simulink model "quad_sim_mult_UAVs_coop_localization"  (R2017a)
settings: Solver=VariableStepAuto  StartTime=0.0  StopTime=60  FixedStep=0.02  MaxStep=0.03  MinStep=0.02  RelTol=1e-3  EnableMultiTasking=on
InitFcn:
  | setup_gains
  | % --- Outer loop gains --------
  | %P_X=9.44;   I_X=0.23;  D_X=2.36;
  | %P_Y=9.33;   I_Y=0.18;  D_Y=1.54;
  | % --------------------------
  | 
  | %CARLA TUNNED PID
  | %P_Z = 51.037;       I_Z = 43.051;        D_Z = 11.771;
  | %P_Z = 0.5;       I_Z = 0.15;        D_Z = 0.2;
  | %P_Z = 32.55;       I_Z = 9.82;        D_Z = 4.65 ;
  | 
  | global clientID;
  | clientID=-1;
values from neighbouring files (symbols this model uses):
  End_POS_coop = Start_POS+0.5    [setup_gains.m]
  Kd_az = 0.001    [setup_gains.m]
  Kd_px = 0.5    [setup_gains.m]
  Kd_py = 0.5    [setup_gains.m]
  Kd_pz = 0.025    [setup_gains.m]
  Kd_vx = 2    [setup_gains.m]
  Kd_vy = 2    [setup_gains.m]
  Kd_vz = 0.05    [setup_gains.m]
  Ki_az = 0.01    [setup_gains.m]
  Ki_px = 0.001    [setup_gains.m]
  Ki_py = 0.001    [setup_gains.m]
  Ki_pz = 0.001    [setup_gains.m]
  Ki_vx = 0.1    [setup_gains.m]
  Ki_vy = 0.1    [setup_gains.m]
  Ki_vz = 2.5    [setup_gains.m]
  Kp_az = 0.75    [setup_gains.m]
  Kp_px = 1    [setup_gains.m]
  Kp_py = 1    [setup_gains.m]
  Kp_pz = 0.5    [setup_gains.m]
  Kp_vx = 15.00    (= 15)    [setup_gains.m]
  Kp_vy = 15.00    (= 15)    [setup_gains.m]
  Kp_vz = 5    [setup_gains.m]
  s1 = cputime()*10    [setup_gains.m]
  s2 = round(s1+randn*10 + 1)    [setup_gains.m]
  s3 = round(s2+randn*10 + 32)    [setup_gains.m]
  s4 = round(s3+randn*10 + 55)    [setup_gains.m]
  Start_POS = [ -1.00 -1.00 1.05 ... (first row only)    [setup_gains.m]
  var_accel = 0.0001    [setup_gains.m]
  var_pos = 0.5^2    (= 0.25)    [setup_gains.m]
  var_ranges = 0.0025    [setup_gains.m]
undefined symbols (not defined in the file or in its folder): W, X, Y, Z
libraries: dspindex x15, robotlib x13, dspsigops x12
(part 1 of 2)
settings Model: Creator=kleber  LastModifiedBy=Cabral
settings DataIOCC: SaveFormat=Array
settings OptimizationCC: LifeSpan=inf
settings DebuggingCC: SolverPrmCheckMsg=warning  SFUnexpectedBacktrackingDiag=warning  SFNoUnconditionalDefaultTransitionDiag=warning  SFExecutionAtInitializationDiag=none
settings HardwareCC: ProdBitPerPointer=32  ProdBitPerSizeT=32  ProdBitPerPtrDiffT=32  ProdLargestAtomicFloat=None  ProdIntDivRoundTo=Undefined  ProdEndianess=Unspecified  ProdWordSize=32  ProdHWDeviceType=32-bit Generic
settings ModelReferenceCC: PropagateSignalLabelsOutOfModel=off
settings GRTTargetCC: TargetLangStandard=C89/C90 (ANSI)  GeneratePreprocessorConditionals=Disable all
settings ConfigComp: CovMetricSettings=dw  CovHtmlReporting=on  CovSaveCumulativeToWorkspaceVar=on  CovSaveSingleToWorkspaceVar=on  CovExternalEMLEnable=off  CovSFcnEnable=off

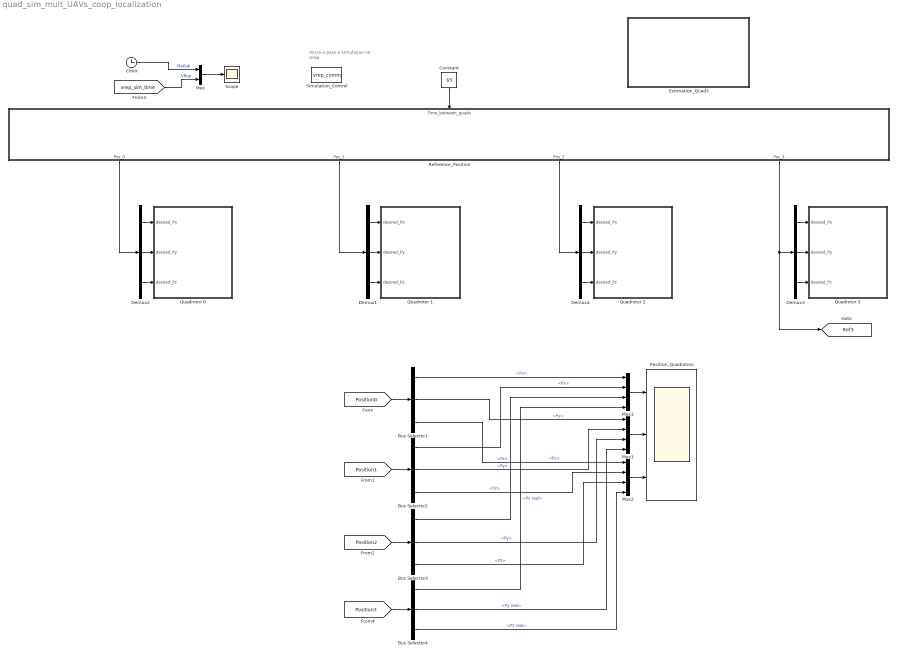
== system quad_sim_mult_UAVs_coop_localization ==
  note: Inicia e para a simulaçao no Vrep
  Bus Selector1 : BusSelector  OutputSignals=Px,Py,Pz
  Bus Selector2 : BusSelector  OutputSignals=Px,Py,Pz
  Bus Selector3 : BusSelector  OutputSignals=Px,Py,Pz
  Bus Selector4 : BusSelector  OutputSignals=Px real,Py real,Pz real
  Clock : Clock
  Constant : Constant  Value=65
  Demux{1..4} (4 alike) : Demux  Outputs=3
  Estimation_Quad3 : Subsystem
  Mux : Mux  Inputs=2
  Mux1 : Mux
  Mux2 : Mux
  Mux3 : Mux
  Position_Quadrotors : Scope  NumInputPorts=3
  Quadrotor 0 : Subsystem
  Quadrotor 1 : Subsystem
  Quadrotor 2 : Subsystem
  Quadrotor 3 : Subsystem
  Reference_Position : Subsystem
  Scope : Scope
  Simulation_Control : S-Function  FunctionName=vrep_comm  SFunctionDeploymentMode=off  EnableBusSupport=off
  tag scope: Ref3=global
  wires:
  Constant/1 -> Reference_Position/1(Time_between_quads)
  Demux1/1 -> Quadrotor 1/1(desired_Px)
  Demux1/2 -> Quadrotor 1/2(desired_Py)
  Demux1/3 -> Quadrotor 1/3(desired_Pz)
  Demux2/1 -> Quadrotor 0/1(desired_Px)
  Demux2/2 -> Quadrotor 0/2(desired_Py)
  Demux2/3 -> Quadrotor 0/3(desired_Pz)
  Reference_Position/1(Pos_0) -> Demux2/1
  Reference_Position/2(Pos_1) -> Demux1/1
  Demux4/1 -> Quadrotor 2/1(desired_Px)
  Demux4/2 -> Quadrotor 2/2(desired_Py)
  Demux4/3 -> Quadrotor 2/3(desired_Pz)
  Reference_Position/3(Pos_2) -> Demux4/1
  Demux3/1 -> Quadrotor 3/1(desired_Px)
  Demux3/2 -> Quadrotor 3/2(desired_Py)
  Demux3/3 -> Quadrotor 3/3(desired_Pz)
  Reference_Position/4(Pos_3) -> [Ref3], Demux3/1
  Mux/1 -> Scope/1
  Clock/1 -> Mux/1  "Matlab"
  [vrep_sim_time] -> Mux/2  "VRep"
  Bus Selector1/1 -> Mux3/1  "<Px>"
  [Position0] -> Bus Selector1/1
  Bus Selector1/2 -> Mux1/1  "<Py>"
  Bus Selector1/3 -> Mux2/1  "<Pz>"
  [Position1] -> Bus Selector2/1
  Bus Selector2/3 -> Mux2/2  "<Pz>"
  Bus Selector2/2 -> Mux1/2  "<Py>"
  Bus Selector2/1 -> Mux3/2  "<Px>"
  [Position2] -> Bus Selector3/1
  Bus Selector3/2 -> Mux1/3  "<Py>"
  Bus Selector3/3 -> Mux2/3  "<Pz>"
  Bus Selector3/1 -> Mux3/3  "<Px>"
  [Position3] -> Bus Selector4/1
  Mux3/1 -> Position_Quadrotors/1
  Mux2/1 -> Position_Quadrotors/3
  Mux1/1 -> Position_Quadrotors/2
  Bus Selector4/1 -> Mux3/4  "<Px real>"
  Bus Selector4/2 -> Mux1/4  "<Py real>"
  Bus Selector4/3 -> Mux2/4  "<Pz real>"

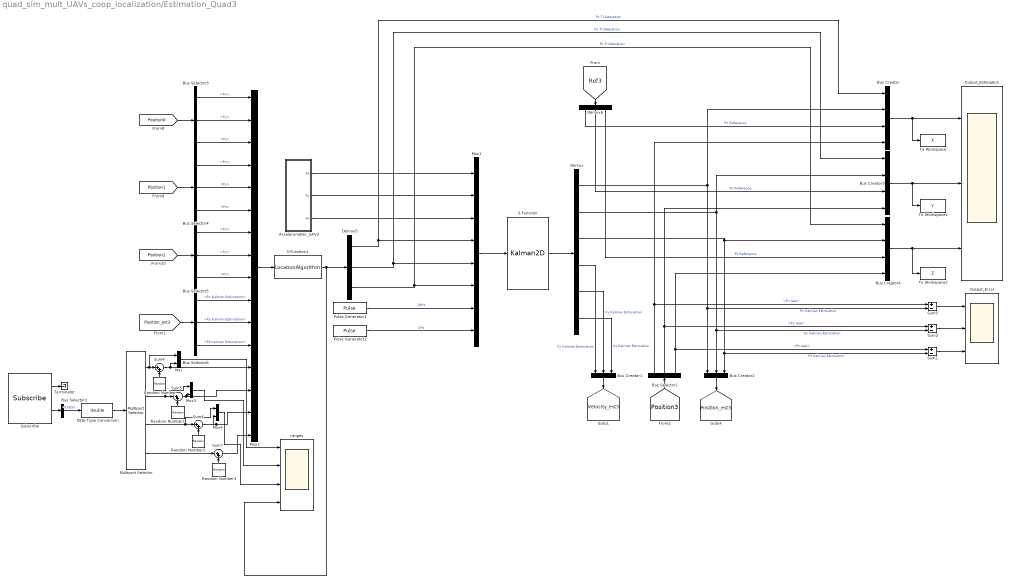
== system quad_sim_mult_UAVs_coop_localization/Estimation_Quad3 ==
  Accelerometer_UAV3 : Subsystem
  Bus Creator : BusCreator  Inputs=4
  Bus Creator1 : BusCreator  Inputs=3
  Bus Creator2 : BusCreator  Inputs=3
  Bus Creator3 : BusCreator  Inputs=4
  Bus Creator4 : BusCreator  Inputs=4
  Bus Selector1 : BusSelector  OutputSignals=Px real,Py real,Pz real
  Bus Selector2 : BusSelector  OutputSignals=Data
  Bus Selector3 : BusSelector  OutputSignals=Px,Py,Pz
  Bus Selector4 : BusSelector  OutputSignals=Px,Py,Pz
  Bus Selector5 : BusSelector  OutputSignals=Px,Py,Pz
  Bus Selector6 : BusSelector  OutputSignals=Px Kalman Estimation,Py Kalman Estimation,Pz Kalman Estimation
  Data Type Conversion : DataTypeConversion  OutDataTypeStr=double
  Demux : Demux  Outputs=6
  Demux5 : Demux  Outputs=3
  Demux6 : Demux  Outputs=3
  Multiport Selector : dspindex/Multiport Selector  rowsOrCols=Rows  idxCellArray={ 3,5,6,7}  idxErrMode=Generate Error
  Mux : Mux  Inputs=2
  Mux1 : Mux  Inputs=8
  Mux2 : Mux  Inputs=16
  Mux3 : Mux  Inputs=2
  Mux4 : Mux  Inputs=2
  Output_Error : Scope  NumInputPorts=3
  Output_Estimation : Scope  NumInputPorts=3
  Pulse Generator1 : DiscretePulseGenerator  PulseType=Time based  Period=0.1  PulseWidth=50
  Pulse Generator2 : DiscretePulseGenerator  PulseType=Time based  Period=1  PulseWidth=50
  Random Number : RandomNumber  Variance=var_ranges  Seed=s1  SampleTime=0.1
  Random Number1 : RandomNumber  Variance=var_ranges  Seed=s2  SampleTime=0.1
  Random Number2 : RandomNumber  Variance=var_ranges  Seed=s3  SampleTime=0.1
  Random Number3 : RandomNumber  Variance=var_ranges  Seed=s4  SampleTime=0.1
  S-Function : S-Function  FunctionName=Kalman2D  SFunctionDeploymentMode=off  EnableBusSupport=off
  S-Function1 : S-Function  FunctionName=LocationAlgorithm  SFunctionDeploymentMode=off  EnableBusSupport=off
  Subscribe : robotlib/Subscribe  SourceLibraryInfo=This block requires Robotics System Toolbox  topicSource=Select from ROS network  topic=/RangeSensors  messageType=std_msgs/Float32MultiArray  sampleTime=-1  messageQueueLength=51
      settings: SourceProductBaseCode=RO
  Sum1 : Sum  Inputs=+-
  Sum2 : Sum  Inputs=+-
  Sum3 : Sum  Inputs=+-
  Sum{4..7} (4 alike) : Sum  Inputs=|++
  Terminator : Terminator
  To Workspace : ToWorkspace  VariableName=X  SaveFormat=Timeseries  SampleTime=-1
  To Workspace1 : ToWorkspace  VariableName=Y  SaveFormat=Timeseries  SampleTime=-1
  To Workspace2 : ToWorkspace  VariableName=Z  SaveFormat=Timeseries  SampleTime=-1
  ranges : Scope  NumInputPorts=4
  tag scope: Position_est3=global, Velocity_est3=global
  wires:
  Bus Selector4/2 -> Mux2/5  "<Py>"
  Multiport Selector/4 -> Sum7/1
  Bus Selector5/3 -> Mux2/9  "<Pz>"
  [Position1] -> Bus Selector4/1
  Random Number3/1 -> Sum7/2
  Random Number/1 -> Sum4/2
  Random Number2/1 -> Sum6/2
  Subscribe/1 -> Terminator/1
  Sum4/1 -> Mux/2, Mux2/13
  Multiport Selector/2 -> Mux3/1, Sum5/1
  Sum5/1 -> Mux3/2, Mux2/14
  Mux2/1 -> S-Function1/1
  Multiport Selector/1 -> Mux/1, Sum4/1
  Bus Selector5/1 -> Mux2/7  "<Px>"
  Bus Selector5/2 -> Mux2/8  "<Py>"
  Sum6/1 -> Mux4/2, Mux2/15
  [Position2] -> Bus Selector5/1
  Random Number1/1 -> Sum5/2
  Bus Selector4/1 -> Mux2/4  "<Px>"
  Bus Selector4/3 -> Mux2/6  "<Pz>"
  Subscribe/2 -> Bus Selector2/1
  S-Function1/1 -> Demux5/1, ranges/4
  Bus Selector3/3 -> Mux2/3  "<Pz>"
  Bus Selector3/2 -> Mux2/2  "<Py>"
  Multiport Selector/3 -> Mux4/1, Sum6/1
  Bus Selector3/1 -> Mux2/1  "<Px>"
  Data Type Conversion/1 -> Multiport Selector/1
  Sum7/1 -> Mux2/16
  Bus Selector2/1 -> Data Type Conversion/1  "<Data>"
  [Position0] -> Bus Selector3/1
  Demux5/2 -> Mux1/5, Bus Creator3/1  "Py Trilateration"
  Demux/1 -> Bus Creator/2, Sum3/2, Bus Creator2/1  "Px Kalman Estimation"
  Demux/2 -> Bus Creator3/2, Sum2/2, Bus Creator2/2  "Py Kalman Estimation"
  Bus Creator/1 -> To Workspace/1, Output_Estimation/1
  Pulse Generator1/1 -> Mux1/7  "10Hz"
  Bus Creator3/1 -> Output_Estimation/2, To Workspace1/1
  Bus Creator4/1 -> To Workspace2/1, Output_Estimation/3
  S-Function/1 -> Demux/1
  Demux5/1 -> Bus Creator/1, Mux1/4  "Px Trilateration"
  Mux1/1 -> S-Function/1
  Pulse Generator2/1 -> Mux1/8  "1Hz"
  Demux5/3 -> Bus Creator4/1, Mux1/6  "Pz Trilateration"
  Demux/3 -> Sum1/2, Bus Creator2/3, Bus Creator4/2  "Pz Kalman Estimation"
  [Position3] -> Bus Selector1/1
  Bus Selector1/1 -> Sum3/1, Bus Creator/4  "<Px real>"
  Bus Selector1/2 -> Bus Creator3/4, Sum2/1  "<Py real>"
  Bus Selector1/3 -> Bus Creator4/4, Sum1/1  "<Pz real>"
  [Ref3] -> Demux6/1
  Demux6/1 -> Bus Creator/3  "Px Reference"
  Demux6/2 -> Bus Creator3/3  "Py Reference"
  Demux6/3 -> Bus Creator4/3  "Pz Reference"
  Bus Creator2/1 -> [Position_est3]
  Accelerometer_UAV3/2(Ay) -> Mux1/2
  Accelerometer_UAV3/3(Az) -> Mux1/3
  Accelerometer_UAV3/1(Ax) -> Mux1/1
  Sum3/1 -> Output_Error/1
  Sum2/1 -> Output_Error/2
  Sum1/1 -> Output_Error/3
  Bus Creator1/1 -> [Velocity_est3]
  Demux/6 -> Bus Creator1/3  "Vz Kalman Estimation"
  Demux/5 -> Bus Creator1/2  "Vy Kalman Estimation"
  Demux/4 -> Bus Creator1/1  "Vx Kalman Estimation"
  Mux4/1 -> ranges/3
  Mux3/1 -> ranges/2
  Mux/1 -> ranges/1
  Bus Selector6/1 -> Mux2/10  "<Px Kalman Estimation>"
  Bus Selector6/2 -> Mux2/11  "<Py Kalman Estimation>"
  Bus Selector6/3 -> Mux2/12  "<Pz Kalman Estimation>"
  [Position_est3] -> Bus Selector6/1

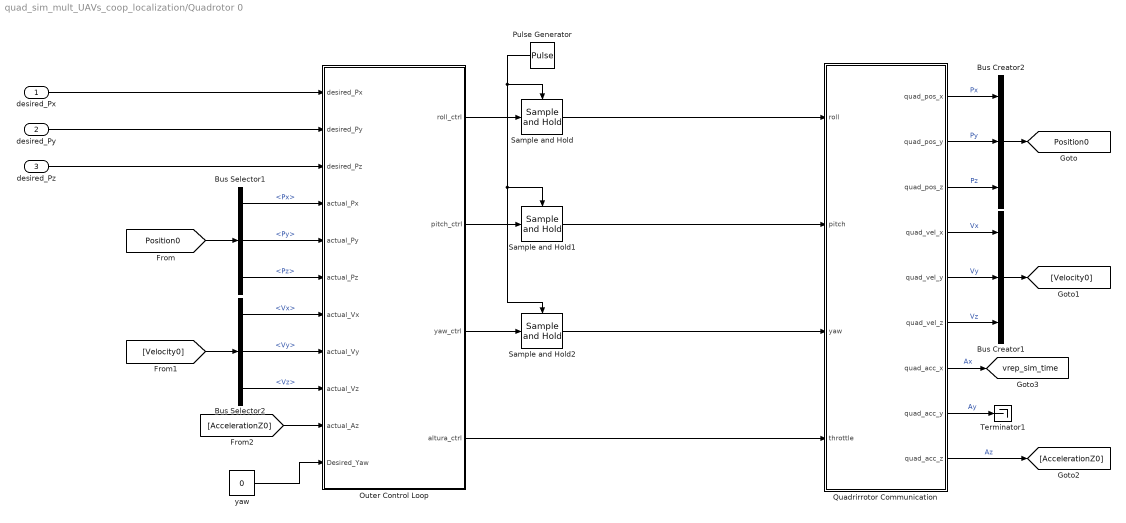
== system quad_sim_mult_UAVs_coop_localization/Quadrotor 0 ==
  desired_Px : Inport
  desired_Py : Inport  Port=2
  desired_Pz : Inport  Port=3
  Bus Creator1 : BusCreator  Inputs=3
  Bus Creator2 : BusCreator  Inputs=3
  Bus Selector1 : BusSelector  OutputSignals=Px,Py,Pz
  Bus Selector2 : BusSelector  OutputSignals=Vx,Vy,Vz
  Outer Control Loop : Subsystem
  Pulse Generator : DiscretePulseGenerator  PulseType=Time based  Period=0.1  PulseWidth=20
  Quadrirrotor Communication : Subsystem
  Sample and Hold : dspsigops/Sample and Hold  trig=Rising edge  initCond=0  latchinput=off
  Sample and Hold1 : dspsigops/Sample and Hold  trig=Rising edge  initCond=0  latchinput=off
  Sample and Hold2 : dspsigops/Sample and Hold  trig=Rising edge  initCond=0  latchinput=off
  Terminator1 : Terminator
  yaw : Constant  Value=0
  tag scope: Position0=global, vrep_sim_time=global
  wires:
  Quadrirrotor Communication/8(quad_acc_y) -> Terminator1/1  "Ay"
  [AccelerationZ0] -> Outer Control Loop/10(actual_Az)
  Quadrirrotor Communication/9(quad_acc_z) -> [AccelerationZ0]  "Az"
  yaw/1 -> Outer Control Loop/11(Desired_Yaw)
  Pulse Generator/1 -> Sample and Hold/Trigger, Sample and Hold1/Trigger, Sample and Hold2/Trigger
  Outer Control Loop/3(yaw_ctrl) -> Sample and Hold2/1
  Outer Control Loop/2(pitch_ctrl) -> Sample and Hold1/1
  Outer Control Loop/1(roll_ctrl) -> Sample and Hold/1
  desired_Py/1 -> Outer Control Loop/2(desired_Py)
  desired_Px/1 -> Outer Control Loop/1(desired_Px)
  desired_Pz/1 -> Outer Control Loop/3(desired_Pz)
  [Position0] -> Bus Selector1/1
  Bus Selector1/3 -> Outer Control Loop/6(actual_Pz)  "<Pz>"
  Bus Selector1/2 -> Outer Control Loop/5(actual_Py)  "<Py>"
  Bus Selector1/1 -> Outer Control Loop/4(actual_Px)  "<Px>"
  Quadrirrotor Communication/4(quad_vel_x) -> Bus Creator1/1  "Vx"
  Quadrirrotor Communication/5(quad_vel_y) -> Bus Creator1/2  "Vy"
  Quadrirrotor Communication/6(quad_vel_z) -> Bus Creator1/3  "Vz"
  Bus Creator1/1 -> [Velocity0]
  Quadrirrotor Communication/3(quad_pos_z) -> Bus Creator2/3  "Pz"
  Quadrirrotor Communication/2(quad_pos_y) -> Bus Creator2/2  "Py"
  Quadrirrotor Communication/1(quad_pos_x) -> Bus Creator2/1  "Px"
  Bus Creator2/1 -> [Position0]
  [Velocity0] -> Bus Selector2/1
  Bus Selector2/3 -> Outer Control Loop/9(actual_Vz)  "<Vz>"
  Bus Selector2/2 -> Outer Control Loop/8(actual_Vy)  "<Vy>"
  Bus Selector2/1 -> Outer Control Loop/7(actual_Vx)  "<Vx>"
  Quadrirrotor Communication/7(quad_acc_x) -> [vrep_sim_time]  "Ax"
  Sample and Hold/1 -> Quadrirrotor Communication/1(roll)
  Sample and Hold1/1 -> Quadrirrotor Communication/2(pitch)
  Sample and Hold2/1 -> Quadrirrotor Communication/3(yaw)
  Outer Control Loop/4(altura_ctrl) -> Quadrirrotor Communication/4(throttle)

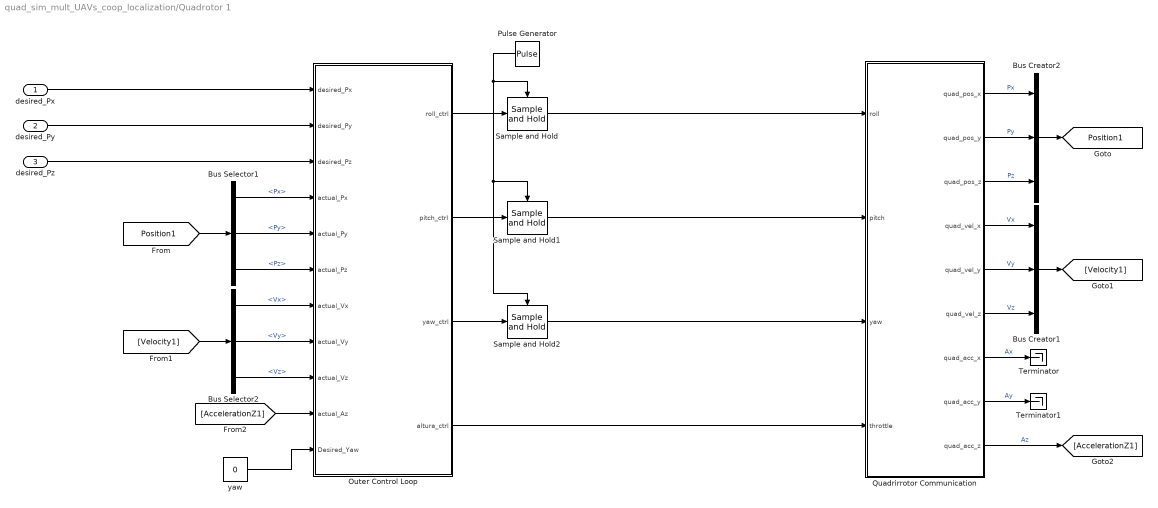
== system quad_sim_mult_UAVs_coop_localization/Quadrotor 1 ==
  desired_Px : Inport
  desired_Py : Inport  Port=2
  desired_Pz : Inport  Port=3
  Bus Creator1 : BusCreator  Inputs=3
  Bus Creator2 : BusCreator  Inputs=3
  Bus Selector1 : BusSelector  OutputSignals=Px,Py,Pz
  Bus Selector2 : BusSelector  OutputSignals=Vx,Vy,Vz
  Outer Control Loop : Subsystem
  Pulse Generator : DiscretePulseGenerator  PulseType=Time based  Period=0.1  PulseWidth=20
  Quadrirrotor Communication : Subsystem
  Sample and Hold : dspsigops/Sample and Hold  trig=Rising edge  initCond=0  latchinput=off
  Sample and Hold1 : dspsigops/Sample and Hold  trig=Rising edge  initCond=0  latchinput=off
  Sample and Hold2 : dspsigops/Sample and Hold  trig=Rising edge  initCond=0  latchinput=off
  Terminator : Terminator
  Terminator1 : Terminator
  yaw : Constant  Value=0
  tag scope: Position1=global
  wires:
  Bus Selector2/1 -> Outer Control Loop/7(actual_Vx)  "<Vx>"
  Bus Selector2/2 -> Outer Control Loop/8(actual_Vy)  "<Vy>"
  Bus Selector2/3 -> Outer Control Loop/9(actual_Vz)  "<Vz>"
  [Velocity1] -> Bus Selector2/1
  Bus Creator2/1 -> [Position1]
  Quadrirrotor Communication/1(quad_pos_x) -> Bus Creator2/1  "Px"
  Quadrirrotor Communication/2(quad_pos_y) -> Bus Creator2/2  "Py"
  Quadrirrotor Communication/3(quad_pos_z) -> Bus Creator2/3  "Pz"
  Bus Creator1/1 -> [Velocity1]
  Quadrirrotor Communication/6(quad_vel_z) -> Bus Creator1/3  "Vz"
  Quadrirrotor Communication/5(quad_vel_y) -> Bus Creator1/2  "Vy"
  Quadrirrotor Communication/4(quad_vel_x) -> Bus Creator1/1  "Vx"
  [Position1] -> Bus Selector1/1
  desired_Px/1 -> Outer Control Loop/1(desired_Px)
  Outer Control Loop/1(roll_ctrl) -> Sample and Hold/1
  Outer Control Loop/2(pitch_ctrl) -> Sample and Hold1/1
  Outer Control Loop/3(yaw_ctrl) -> Sample and Hold2/1
  Pulse Generator/1 -> Sample and Hold2/Trigger, Sample and Hold1/Trigger, Sample and Hold/Trigger
  yaw/1 -> Outer Control Loop/11(Desired_Yaw)
  Quadrirrotor Communication/9(quad_acc_z) -> [AccelerationZ1]  "Az"
  [AccelerationZ1] -> Outer Control Loop/10(actual_Az)
  Quadrirrotor Communication/8(quad_acc_y) -> Terminator1/1  "Ay"
  Quadrirrotor Communication/7(quad_acc_x) -> Terminator/1  "Ax"
  Bus Selector1/1 -> Outer Control Loop/4(actual_Px)  "<Px>"
  desired_Pz/1 -> Outer Control Loop/3(desired_Pz)
  desired_Py/1 -> Outer Control Loop/2(desired_Py)
  Bus Selector1/2 -> Outer Control Loop/5(actual_Py)  "<Py>"
  Bus Selector1/3 -> Outer Control Loop/6(actual_Pz)  "<Pz>"
  Sample and Hold/1 -> Quadrirrotor Communication/1(roll)
  Sample and Hold1/1 -> Quadrirrotor Communication/2(pitch)
  Sample and Hold2/1 -> Quadrirrotor Communication/3(yaw)
  Outer Control Loop/4(altura_ctrl) -> Quadrirrotor Communication/4(throttle)

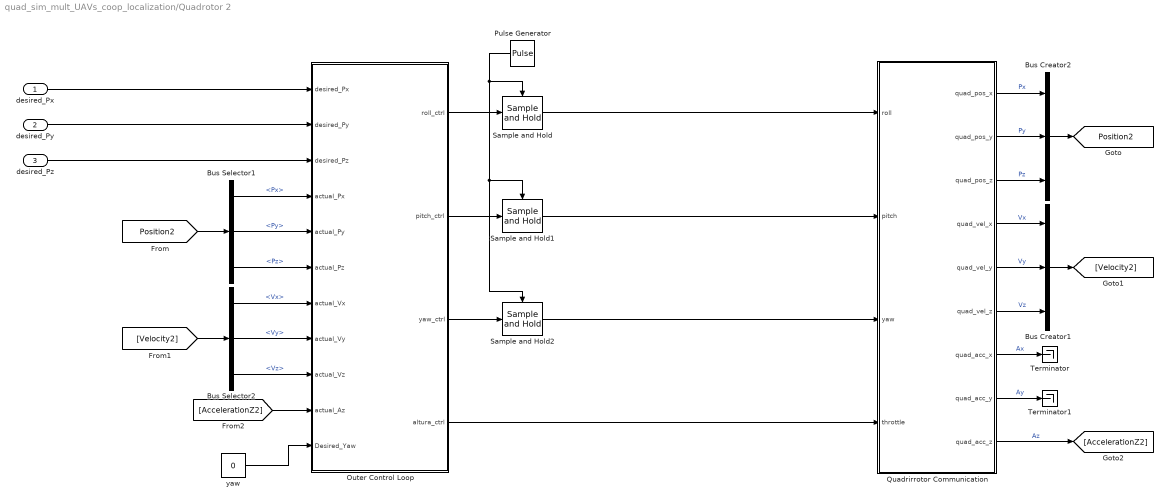
== system quad_sim_mult_UAVs_coop_localization/Quadrotor 2 ==
  desired_Px : Inport
  desired_Py : Inport  Port=2
  desired_Pz : Inport  Port=3
  Bus Creator1 : BusCreator  Inputs=3
  Bus Creator2 : BusCreator  Inputs=3
  Bus Selector1 : BusSelector  OutputSignals=Px,Py,Pz
  Bus Selector2 : BusSelector  OutputSignals=Vx,Vy,Vz
  Outer Control Loop : Subsystem
  Pulse Generator : DiscretePulseGenerator  PulseType=Time based  Period=0.1  PulseWidth=20
  Quadrirrotor Communication : Subsystem
  Sample and Hold : dspsigops/Sample and Hold  trig=Rising edge  initCond=0  latchinput=off
  Sample and Hold1 : dspsigops/Sample and Hold  trig=Rising edge  initCond=0  latchinput=off
  Sample and Hold2 : dspsigops/Sample and Hold  trig=Rising edge  initCond=0  latchinput=off
  Terminator : Terminator
  Terminator1 : Terminator
  yaw : Constant  Value=0
  tag scope: Position2=global
  wires:
  Quadrirrotor Communication/7(quad_acc_x) -> Terminator/1  "Ax"
  Quadrirrotor Communication/8(quad_acc_y) -> Terminator1/1  "Ay"
  [AccelerationZ2] -> Outer Control Loop/10(actual_Az)
  Quadrirrotor Communication/9(quad_acc_z) -> [AccelerationZ2]  "Az"
  yaw/1 -> Outer Control Loop/11(Desired_Yaw)
  Pulse Generator/1 -> Sample and Hold/Trigger, Sample and Hold1/Trigger, Sample and Hold2/Trigger
  Outer Control Loop/3(yaw_ctrl) -> Sample and Hold2/1
  Outer Control Loop/2(pitch_ctrl) -> Sample and Hold1/1
  Outer Control Loop/1(roll_ctrl) -> Sample and Hold/1
  desired_Px/1 -> Outer Control Loop/1(desired_Px)
  [Position2] -> Bus Selector1/1
  Quadrirrotor Communication/4(quad_vel_x) -> Bus Creator1/1  "Vx"
  Quadrirrotor Communication/5(quad_vel_y) -> Bus Creator1/2  "Vy"
  Quadrirrotor Communication/6(quad_vel_z) -> Bus Creator1/3  "Vz"
  Bus Creator1/1 -> [Velocity2]
  Quadrirrotor Communication/3(quad_pos_z) -> Bus Creator2/3  "Pz"
  Quadrirrotor Communication/2(quad_pos_y) -> Bus Creator2/2  "Py"
  Quadrirrotor Communication/1(quad_pos_x) -> Bus Creator2/1  "Px"
  Bus Creator2/1 -> [Position2]
  [Velocity2] -> Bus Selector2/1
  Bus Selector2/3 -> Outer Control Loop/9(actual_Vz)  "<Vz>"
  Bus Selector2/2 -> Outer Control Loop/8(actual_Vy)  "<Vy>"
  Bus Selector2/1 -> Outer Control Loop/7(actual_Vx)  "<Vx>"
  Bus Selector1/1 -> Outer Control Loop/4(actual_Px)  "<Px>"
  desired_Pz/1 -> Outer Control Loop/3(desired_Pz)
  desired_Py/1 -> Outer Control Loop/2(desired_Py)
  Bus Selector1/2 -> Outer Control Loop/5(actual_Py)  "<Py>"
  Bus Selector1/3 -> Outer Control Loop/6(actual_Pz)  "<Pz>"
  Sample and Hold/1 -> Quadrirrotor Communication/1(roll)
  Sample and Hold1/1 -> Quadrirrotor Communication/2(pitch)
  Sample and Hold2/1 -> Quadrirrotor Communication/3(yaw)
  Outer Control Loop/4(altura_ctrl) -> Quadrirrotor Communication/4(throttle)

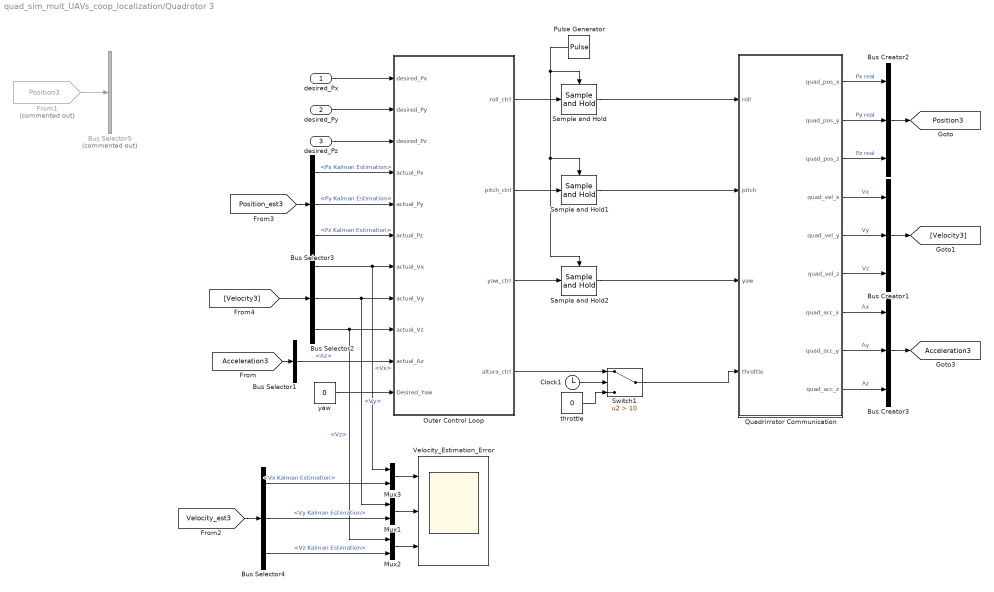
== system quad_sim_mult_UAVs_coop_localization/Quadrotor 3 ==
  desired_Px : Inport
  desired_Py : Inport  Port=2
  desired_Pz : Inport  Port=3
  Bus Creator1 : BusCreator  Inputs=3
  Bus Creator2 : BusCreator  Inputs=3
  Bus Creator3 : BusCreator  Inputs=3
  Bus Selector1 : BusSelector  OutputSignals=Az
  Bus Selector2 : BusSelector  OutputSignals=Vx,Vy,Vz
  Bus Selector3 : BusSelector  OutputSignals=Px Kalman Estimation,Py Kalman Estimation,Pz Kalman Estimation
  Bus Selector4 : BusSelector  OutputSignals=Vx Kalman Estimation,Vy Kalman Estimation,Vz Kalman Estimation
  Bus Selector5 : BusSelector  Commented=on  OutputSignals=Px real,Py real,Pz real
  Clock1 : Clock
  From1 : From  Commented=on  GotoTag=Position3  TagVisibility=global
  Mux1 : Mux  Inputs=2
  Mux2 : Mux  Inputs=2
  Mux3 : Mux  Inputs=2
  Outer Control Loop : Subsystem
  Pulse Generator : DiscretePulseGenerator  PulseType=Time based  Period=0.1  PulseWidth=20
  Quadrirrotor Communication : Subsystem
  Sample and Hold : dspsigops/Sample and Hold  trig=Rising edge  initCond=0  latchinput=off
  Sample and Hold1 : dspsigops/Sample and Hold  trig=Rising edge  initCond=0  latchinput=off
  Sample and Hold2 : dspsigops/Sample and Hold  trig=Rising edge  initCond=0  latchinput=off
  Switch1 : Switch  Criteria=u2 > Threshold  Threshold=10
  Velocity_Estimation_Error : Scope  NumInputPorts=3
  throttle : Constant  Value=0
  yaw : Constant  Value=0
  tag scope: Acceleration3=global, Position3=global
  wires:
  desired_Py/1 -> Outer Control Loop/2(desired_Py)
  desired_Pz/1 -> Outer Control Loop/3(desired_Pz)
  Bus Selector2/1 -> Outer Control Loop/7(actual_Vx), Mux3/1  "<Vx>"
  Bus Selector2/2 -> Mux1/1, Outer Control Loop/8(actual_Vy)  "<Vy>"
  Bus Selector2/3 -> Mux2/1, Outer Control Loop/9(actual_Vz)  "<Vz>"
  Bus Creator2/1 -> [Position3]
  Quadrirrotor Communication/1(quad_pos_x) -> Bus Creator2/1  "Px real"
  Quadrirrotor Communication/2(quad_pos_y) -> Bus Creator2/2  "Py real"
  Quadrirrotor Communication/3(quad_pos_z) -> Bus Creator2/3  "Pz real"
  Bus Creator1/1 -> [Velocity3]
  Quadrirrotor Communication/6(quad_vel_z) -> Bus Creator1/3  "Vz"
  Quadrirrotor Communication/5(quad_vel_y) -> Bus Creator1/2  "Vy"
  Quadrirrotor Communication/4(quad_vel_x) -> Bus Creator1/1  "Vx"
  desired_Px/1 -> Outer Control Loop/1(desired_Px)
  Outer Control Loop/1(roll_ctrl) -> Sample and Hold/1
  Outer Control Loop/2(pitch_ctrl) -> Sample and Hold1/1
  Outer Control Loop/3(yaw_ctrl) -> Sample and Hold2/1
  Pulse Generator/1 -> Sample and Hold2/Trigger, Sample and Hold1/Trigger, Sample and Hold/Trigger
  yaw/1 -> Outer Control Loop/11(Desired_Yaw)
  Quadrirrotor Communication/9(quad_acc_z) -> Bus Creator3/3  "Az"
  Quadrirrotor Communication/8(quad_acc_y) -> Bus Creator3/2  "Ay"
  Quadrirrotor Communication/7(quad_acc_x) -> Bus Creator3/1  "Ax"
  Sample and Hold/1 -> Quadrirrotor Communication/1(roll)
  Sample and Hold1/1 -> Quadrirrotor Communication/2(pitch)
  Sample and Hold2/1 -> Quadrirrotor Communication/3(yaw)
  Outer Control Loop/4(altura_ctrl) -> Switch1/1
  Bus Creator3/1 -> [Acceleration3]
  [Position_est3] -> Bus Selector3/1
  Clock1/1 -> Switch1/2
  throttle/1 -> Switch1/3
  Switch1/1 -> Quadrirrotor Communication/4(throttle)
  [Acceleration3] -> Bus Selector1/1
  Bus Selector1/1 -> Outer Control Loop/10(actual_Az)  "<Az>"
  Mux3/1 -> Velocity_Estimation_Error/1
  Bus Selector4/1 -> Mux3/2  "<Vx Kalman Estimation>"
  Mux1/1 -> Velocity_Estimation_Error/2
  Bus Selector4/2 -> Mux1/2  "<Vy Kalman Estimation>"
  Mux2/1 -> Velocity_Estimation_Error/3
  Bus Selector4/3 -> Mux2/2  "<Vz Kalman Estimation>"
  [Velocity_est3] -> Bus Selector4/1
  [Velocity3] -> Bus Selector2/1
  From1/1 -> Bus Selector5/1
  Bus Selector3/1 -> Outer Control Loop/4(actual_Px)  "<Px Kalman Estimation>"
  Bus Selector3/2 -> Outer Control Loop/5(actual_Py)  "<Py Kalman Estimation>"
  Bus Selector3/3 -> Outer Control Loop/6(actual_Pz)  "<Pz Kalman Estimation>"

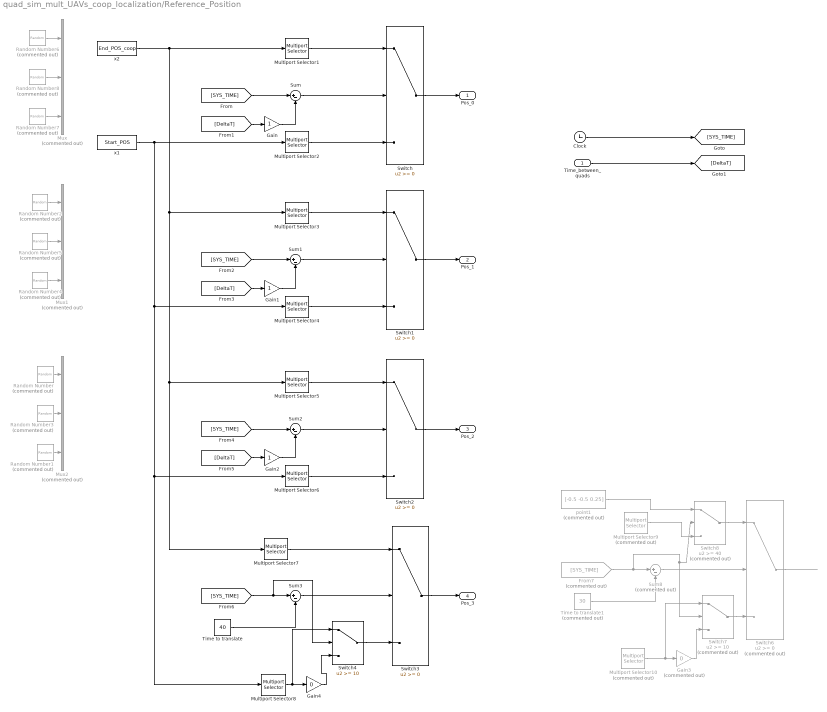
== system quad_sim_mult_UAVs_coop_localization/Reference_Position ==
  Time_between_quads : Inport
  Clock : Clock
  From7 : From  Commented=on  GotoTag=SYS_TIME
  Gain : Gain
  Gain1 : Gain
  Gain2 : Gain
  Gain3 : Gain  Commented=on  Gain=0
  Gain4 : Gain  Gain=0
  Multiport Selector1 : dspindex/Multiport Selector  rowsOrCols=Rows  idxCellArray={1}  idxErrMode=Generate Error
  Multiport Selector10 : dspindex/Multiport Selector  Commented=on  rowsOrCols=Rows  idxCellArray={4}  idxErrMode=Generate Error
  Multiport Selector2 : dspindex/Multiport Selector  rowsOrCols=Rows  idxCellArray={1}  idxErrMode=Generate Error
  Multiport Selector3 : dspindex/Multiport Selector  rowsOrCols=Rows  idxCellArray={2}  idxErrMode=Generate Error
  Multiport Selector4 : dspindex/Multiport Selector  rowsOrCols=Rows  idxCellArray={2}  idxErrMode=Generate Error
  Multiport Selector5 : dspindex/Multiport Selector  rowsOrCols=Rows  idxCellArray={3}  idxErrMode=Generate Error
  Multiport Selector6 : dspindex/Multiport Selector  rowsOrCols=Rows  idxCellArray={3}  idxErrMode=Generate Error
  Multiport Selector7 : dspindex/Multiport Selector  rowsOrCols=Rows  idxCellArray={4}  idxErrMode=Generate Error
  Multiport Selector8 : dspindex/Multiport Selector  rowsOrCols=Rows  idxCellArray={4}  idxErrMode=Generate Error
  Multiport Selector9 : dspindex/Multiport Selector  Commented=on  rowsOrCols=Rows  idxCellArray={4}  idxErrMode=Generate Error
  Mux : Mux  Commented=on  Inputs=3
  Mux1 : Mux  Commented=on  Inputs=3
  Mux2 : Mux  Commented=on  Inputs=3
  Random Number : RandomNumber  Commented=on  Variance=var_pos  Seed=s1  SampleTime=15
  Random Number1 : RandomNumber  Commented=on  Variance=var_pos  Seed=s3  SampleTime=15
  Random Number2 : RandomNumber  Commented=on  Variance=var_pos  Seed=s1*2  SampleTime=15
  Random Number3 : RandomNumber  Commented=on  Variance=var_pos  Seed=s2  SampleTime=15
  Random Number4 : RandomNumber  Commented=on  Variance=var_pos  Seed=s3*2  SampleTime=15
  Random Number5 : RandomNumber  Commented=on  Variance=var_pos  Seed=s2*2  SampleTime=15
  Random Number6 : RandomNumber  Commented=on  Variance=var_pos  Seed=s1*3  SampleTime=15
  Random Number7 : RandomNumber  Commented=on  Variance=var_pos  Seed=s3*3  SampleTime=15
  Random Number8 : RandomNumber  Commented=on  Variance=var_pos  Seed=s2*3  SampleTime=15
  Sum{,1..3} (4 alike) : Sum  Inputs=|+-
  Sum8 : Sum  Commented=on  Inputs=|+-
  Switch{,1..3} (4 alike) : Switch
  Switch4 : Switch  Threshold=10
  Switch6 : Switch  Commented=on
  Switch7 : Switch  Commented=on  Threshold=10
  Switch8 : Switch  Commented=on  Threshold=40
  Time to translate : Constant  Value=40
  Time to translate1 : Constant  Commented=on  Value=30
  point1 : Constant  Commented=on  Value=[-0.5 -0.5 0.25]
  x1 : Constant  Value=Start_POS
  x2 : Constant  Value=End_POS_coop
  Pos_0 : Outport
  Pos_1 : Outport  Port=2
  Pos_2 : Outport  Port=3
  Pos_3 : Outport  Port=4
  wires:
  Switch/1 -> Pos_0/1
  Clock/1 -> [SYS_TIME]
  Time_between_quads/1 -> [DeltaT]
  [DeltaT] -> Gain/1
  Gain/1 -> Sum/2
  [SYS_TIME] -> Sum/1
  Sum1/1 -> Switch1/2
  [SYS_TIME] -> Sum1/1
  Gain1/1 -> Sum1/2
  [DeltaT] -> Gain1/1
  Switch1/1 -> Pos_1/1
  Switch2/1 -> Pos_2/1
  [DeltaT] -> Gain2/1
  Gain2/1 -> Sum2/2
  [SYS_TIME] -> Sum2/1
  Sum/1 -> Switch/2
  Sum2/1 -> Switch2/2
  Switch3/1 -> Pos_3/1
  [SYS_TIME] -> Switch4/2, Sum3/1
  x2/1 -> Multiport Selector7/1, Multiport Selector5/1, Multiport Selector3/1, Multiport Selector1/1
  Sum3/1 -> Switch3/2
  Gain4/1 -> Switch4/3
  Multiport Selector8/1 -> Gain4/1, Switch4/1
  Switch4/1 -> Switch3/3
  Time to translate/1 -> Sum3/2
  point1/1 -> Switch8/1
  Multiport Selector9/1 -> Switch8/3
  Switch8/1 -> Switch6/1
  Time to translate1/1 -> Sum8/2
  Switch7/1 -> Switch6/3
  Multiport Selector10/1 -> Gain3/1, Switch7/1
  Gain3/1 -> Switch7/3
  Sum8/1 -> Switch6/2
  From7/1 -> Sum8/1, Switch7/2, Switch8/2
  Switch6/1 -> ?
  Random Number8/1 -> Mux/2
  Random Number7/1 -> Mux/3
  Random Number6/1 -> Mux/1
  Random Number2/1 -> Mux1/1
  Random Number5/1 -> Mux1/2
  Random Number/1 -> Mux2/1
  Random Number3/1 -> Mux2/2
  Random Number1/1 -> Mux2/3
  Random Number4/1 -> Mux1/3
  x1/1 -> Multiport Selector4/1, Multiport Selector6/1, Multiport Selector8/1, Multiport Selector2/1
  Multiport Selector7/1 -> Switch3/1
  Multiport Selector1/1 -> Switch/1
  Multiport Selector6/1 -> Switch2/3
  Multiport Selector3/1 -> Switch1/1
  Multiport Selector4/1 -> Switch1/3
  Multiport Selector2/1 -> Switch/3
  Multiport Selector5/1 -> Switch2/1

== system quad_sim_mult_UAVs_coop_localization/Estimation_Quad3/Accelerometer_UAV3 ==
  Bus Selector2 : BusSelector  OutputSignals=Ax,Ay,Az
  Mux : Mux  Commented=on
  Random Number : RandomNumber  Variance=var_accel  Seed=s1  SampleTime=0.1
  Random Number1 : RandomNumber  Variance=var_accel  Seed=s3  SampleTime=0.1
  Random Number2 : RandomNumber  Variance=var_accel  Seed=s1*2  SampleTime=0.1
  Random Number3 : RandomNumber  Variance=0.0001  Seed=s2  SampleTime=10
  Random Number4 : RandomNumber  Variance=0.0001  Seed=s4  SampleTime=10
  Random Number5 : RandomNumber  Variance=0.0001  Seed=s2*2  SampleTime=10
  Scope : Scope  Commented=on
  Sum1 : Sum  Inputs=+++
  Sum2 : Sum  Inputs=+++
  Sum3 : Sum  Inputs=+++
  Ax : Outport
  Ay : Outport  Port=2
  Az : Outport  Port=3
  wires:
  Bus Selector2/1 -> Sum3/2  "<Ax>"
  Bus Selector2/3 -> Sum1/2  "<Az>"
  Random Number/1 -> Mux/2, Sum3/1, Mux/1
  Random Number1/1 -> Sum2/1
  Bus Selector2/2 -> Sum2/2  "<Ay>"
  Random Number5/1 -> Sum1/3
  Random Number4/1 -> Sum2/3
  [Acceleration3] -> Bus Selector2/1
  Random Number2/1 -> Sum1/1
  Random Number3/1 -> Mux/3, Sum3/3
  Sum3/1 -> Mux/4, Ax/1
  Sum2/1 -> Ay/1
  Sum1/1 -> Az/1
  Mux/1 -> Scope/1

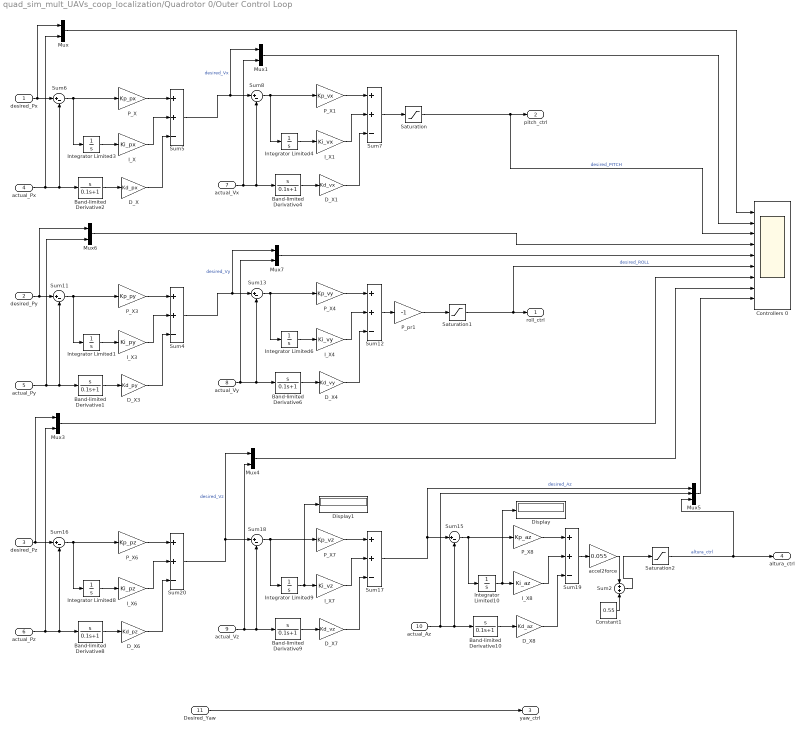
== system quad_sim_mult_UAVs_coop_localization/Quadrotor 0/Outer Control Loop ==
  desired_Px : Inport
  desired_Py : Inport  Port=2
  desired_Pz : Inport  Port=3
  actual_Px : Inport  Port=4
  actual_Py : Inport  Port=5
  actual_Pz : Inport  Port=6
  actual_Vx : Inport  Port=7
  actual_Vy : Inport  Port=8
  actual_Vz : Inport  Port=9
  actual_Az : Inport  Port=10
  Desired_Yaw : Inport  Port=11
  Band-limited Derivative{1..2,4,6,8..10} (7 alike) : TransferFcn  Numerator=[1 0]  Denominator=[0.1 1]
  Constant1 : Constant  Value=0.55
  Controllers 0 : Scope  NumInputPorts=9
  D_X : Gain  Gain=Kd_px
  D_X1 : Gain  Gain=Kd_vx
  D_X3 : Gain  Gain=Kd_py
  D_X4 : Gain  Gain=Kd_vy
  D_X6 : Gain  Gain=Kd_pz
  D_X7 : Gain  Gain=Kd_vz
  D_X8 : Gain  Gain=Kd_az
  Display : Display
  Display1 : Display
  I_X : Gain  Gain=Ki_px
  I_X1 : Gain  Gain=Ki_vx
  I_X3 : Gain  Gain=Ki_py
  I_X4 : Gain  Gain=Ki_vy
  I_X6 : Gain  Gain=Ki_pz
  I_X7 : Gain  Gain=Ki_vz
  I_X8 : Gain  Gain=Ki_az
  Integrator Limited{1,3..4,6} (4 alike) : Integrator  LimitOutput=on  UpperSaturationLimit=100  LowerSaturationLimit=-100
  Integrator Limited10 : Integrator  LimitOutput=on  UpperSaturationLimit=1000  LowerSaturationLimit=-1000
  Integrator Limited8 : Integrator  LimitOutput=on  UpperSaturationLimit=1000  LowerSaturationLimit=-1000
  Integrator Limited9 : Integrator  LimitOutput=on  UpperSaturationLimit=1000  LowerSaturationLimit=-1000
  Mux{,1,3..4,6..7} (6 alike) : Mux  Inputs=2
  Mux5 : Mux  Inputs=3
  P_X : Gain  Gain=Kp_px
  P_X1 : Gain  Gain=Kp_vx
  P_X3 : Gain  Gain=Kp_py
  P_X4 : Gain  Gain=Kp_vy
  P_X6 : Gain  Gain=Kp_pz
  P_X7 : Gain  Gain=Kp_vz
  P_X8 : Gain  Gain=Kp_az
  P_pr1 : Gain  Gain=-1
  Saturation : Saturate  UpperLimit=5  LowerLimit=-5
  Saturation1 : Saturate  UpperLimit=5  LowerLimit=-5
  Saturation2 : Saturate  UpperLimit=10  LowerLimit=0
  Sum{6,8,11,13,15..16,18} (7 alike) : Sum  Inputs=|+-
  Sum{4..5,7,12,17,19..20} (7 alike) : Sum  Inputs=++-
  Sum2 : Sum  Inputs=+|+
  accel2force : Gain  Gain=0.055
  roll_ctrl : Outport
  pitch_ctrl : Outport  Port=2
  yaw_ctrl : Outport  Port=3
  altura_ctrl : Outport  Port=4
  wires:
  Desired_Yaw/1 -> yaw_ctrl/1
  Sum6/1 -> Integrator Limited3/1, P_X/1
  Integrator Limited3/1 -> I_X/1
  P_X/1 -> Sum5/1
  D_X/1 -> Sum5/3
  actual_Px/1 -> Mux/2, Band-limited Derivative2/1, Sum6/2
  Band-limited Derivative2/1 -> D_X/1
  I_X/1 -> Sum5/2
  Saturation2/1 -> Mux5/3, altura_ctrl/1  "altura_ctrl"
  Sum8/1 -> P_X1/1, Integrator Limited4/1
  Integrator Limited4/1 -> I_X1/1
  P_X1/1 -> Sum7/1
  D_X1/1 -> Sum7/3
  actual_Vx/1 -> Mux1/2, Sum8/2, Band-limited Derivative4/1
  Band-limited Derivative4/1 -> D_X1/1
  I_X1/1 -> Sum7/2
  Sum5/1 -> Mux1/1, Sum8/1  "desired_Vx"
  Sum7/1 -> Saturation/1
  Sum11/1 -> P_X3/1, Integrator Limited1/1
  Integrator Limited1/1 -> I_X3/1
  P_X3/1 -> Sum4/1
  D_X3/1 -> Sum4/3
  Band-limited Derivative1/1 -> D_X3/1
  I_X3/1 -> Sum4/2
  Sum13/1 -> Integrator Limited6/1, P_X4/1
  Integrator Limited6/1 -> I_X4/1
  P_X4/1 -> Sum12/1
  D_X4/1 -> Sum12/3
  Band-limited Derivative6/1 -> D_X4/1
  I_X4/1 -> Sum12/2
  Sum4/1 -> Sum13/1, Mux7/1  "desired_Vy"
  Sum12/1 -> P_pr1/1
  Sum16/1 -> Integrator Limited8/1, P_X6/1
  Integrator Limited8/1 -> I_X6/1
  P_X6/1 -> Sum20/1
  D_X6/1 -> Sum20/3
  actual_Pz/1 -> Mux3/2, Band-limited Derivative8/1, Sum16/2
  Band-limited Derivative8/1 -> D_X6/1
  I_X6/1 -> Sum20/2
  Sum18/1 -> P_X7/1, Integrator Limited9/1
  Integrator Limited9/1 -> Display1/1, I_X7/1
  P_X7/1 -> Sum17/1
  D_X7/1 -> Sum17/3
  Band-limited Derivative9/1 -> D_X7/1
  I_X7/1 -> Sum17/2
  Sum15/1 -> Integrator Limited10/1, P_X8/1
  Integrator Limited10/1 -> Display/1, I_X8/1
  P_X8/1 -> Sum19/1
  D_X8/1 -> Sum19/3
  Band-limited Derivative10/1 -> D_X8/1
  I_X8/1 -> Sum19/2
  Mux/1 -> Controllers 0/1
  Mux1/1 -> Controllers 0/2
  actual_Vz/1 -> Mux4/2, Sum18/2, Band-limited Derivative9/1
  Sum20/1 -> Mux4/1, Sum18/1  "desired_Vz"
  actual_Az/1 -> Mux5/2, Band-limited Derivative10/1, Sum15/2
  Sum17/1 -> Mux5/1, Sum15/1  "desired_Az"
  Mux3/1 -> Controllers 0/7
  Mux4/1 -> Controllers 0/8
  Sum19/1 -> accel2force/1
  accel2force/1 -> Sum2/1
  Constant1/1 -> Sum2/2
  desired_Py/1 -> Mux6/1, Sum11/1
  actual_Vy/1 -> Band-limited Derivative6/1, Sum13/2, Mux7/2
  Mux6/1 -> Controllers 0/4
  Mux7/1 -> Controllers 0/5
  P_pr1/1 -> Saturation1/1
  Saturation/1 -> Controllers 0/3, pitch_ctrl/1  "desired_PITCH"
  Mux5/1 -> Controllers 0/9
  Saturation1/1 -> Controllers 0/6, roll_ctrl/1  "desired_ROLL"
  desired_Pz/1 -> Mux3/1, Sum16/1
  Sum2/1 -> Saturation2/1
  desired_Px/1 -> Mux/1, Sum6/1
  actual_Py/1 -> Sum11/2, Band-limited Derivative1/1, Mux6/2

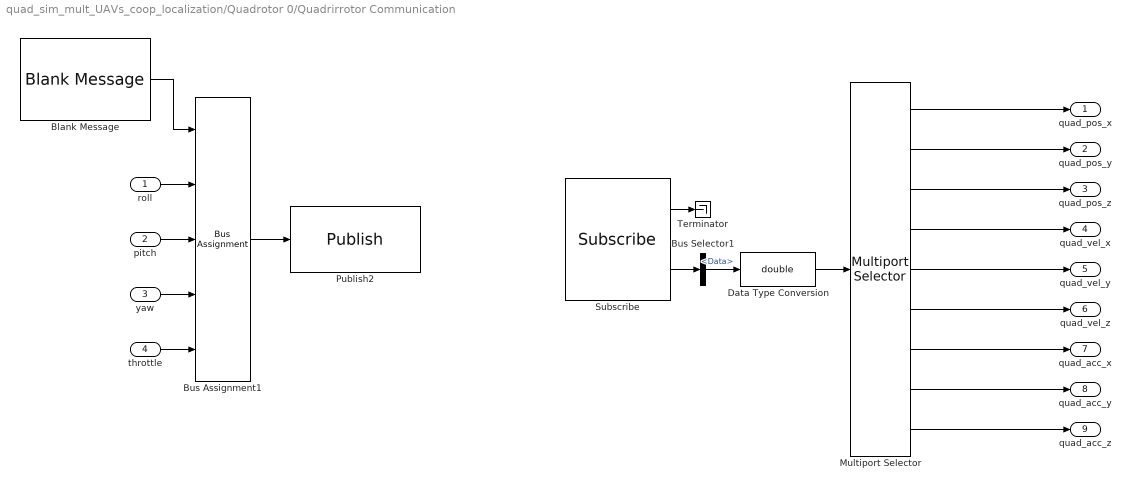
== system quad_sim_mult_UAVs_coop_localization/Quadrotor 0/Quadrirrotor Communication ==
  roll : Inport
  pitch : Inport  Port=2
  yaw : Inport  Port=3
  throttle : Inport  Port=4
  Blank Message : robotlib/Blank Message  SourceLibraryInfo=This block requires Robotics System Toolbox  messageType=geometry_msgs/Quaternion  SampleTime=inf
      settings: SourceProductBaseCode=RO
  Bus Assignment1 : BusAssignment  DialogController=Simulink.DDGSource_BusAssignment  AssignedSignals=X,Y,Z,W
  Bus Selector1 : BusSelector  OutputSignals=Data
  Data Type Conversion : DataTypeConversion  OutDataTypeStr=double
  Multiport Selector : dspindex/Multiport Selector  rowsOrCols=Rows  idxCellArray={ 1,2,3,4,5,6,7,8,9}  idxErrMode=Generate Error
  Publish2 : robotlib/Publish  SourceLibraryInfo=This block requires Robotics System Toolbox  topicSource=Specify your own  topic=/commands_attitude_0  messageType=geometry_msgs/Quaternion  messageQueueLength=105
      settings: SourceProductBaseCode=RO
  Subscribe : robotlib/Subscribe  SourceLibraryInfo=This block requires Robotics System Toolbox  topicSource=Specify your own  topic=/quadrotor_states_0  messageType=std_msgs/Float32MultiArray  sampleTime=-1  messageQueueLength=51
      settings: SourceProductBaseCode=RO
  Terminator : Terminator
  quad_pos_x : Outport
  quad_pos_y : Outport  Port=2
  quad_pos_z : Outport  Port=3
  quad_vel_x : Outport  Port=4
  quad_vel_y : Outport  Port=5
  quad_vel_z : Outport  Port=6
  quad_acc_x : Outport  Port=7
  quad_acc_y : Outport  Port=8
  quad_acc_z : Outport  Port=9
  wires:
  Blank Message/1 -> Bus Assignment1/1
  Subscribe/1 -> Terminator/1
  Subscribe/2 -> Bus Selector1/1
  Bus Assignment1/1 -> Publish2/1
  Multiport Selector/1 -> quad_pos_x/1
  Multiport Selector/2 -> quad_pos_y/1
  Multiport Selector/3 -> quad_pos_z/1
  Multiport Selector/4 -> quad_vel_x/1
  Multiport Selector/5 -> quad_vel_y/1
  Multiport Selector/6 -> quad_vel_z/1
  Multiport Selector/7 -> quad_acc_x/1
  Multiport Selector/8 -> quad_acc_y/1
  Multiport Selector/9 -> quad_acc_z/1
  Data Type Conversion/1 -> Multiport Selector/1
  Bus Selector1/1 -> Data Type Conversion/1  "<Data>"
  throttle/1 -> Bus Assignment1/5
  yaw/1 -> Bus Assignment1/4
  pitch/1 -> Bus Assignment1/3
  roll/1 -> Bus Assignment1/2

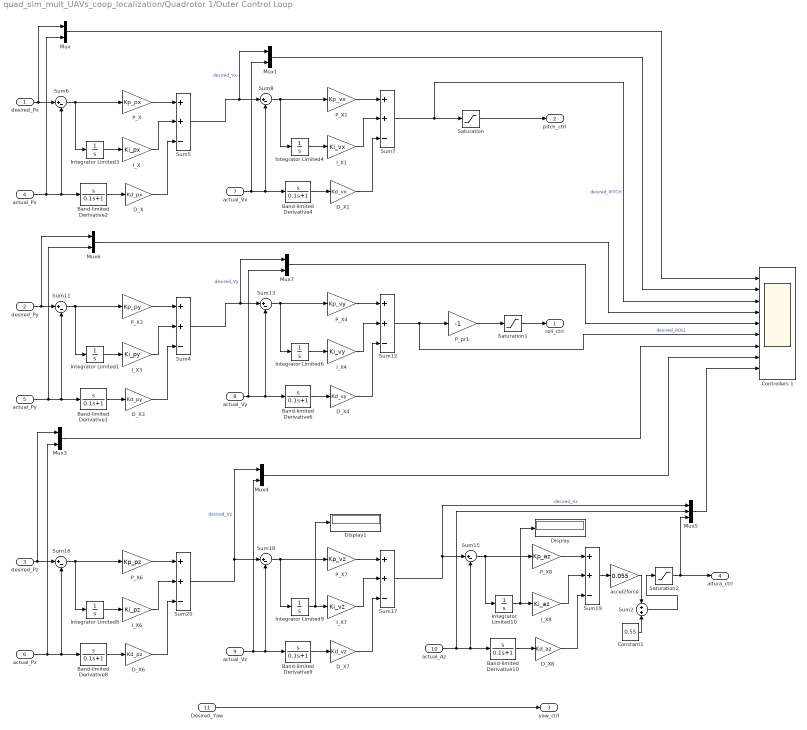
== system quad_sim_mult_UAVs_coop_localization/Quadrotor 1/Outer Control Loop ==
  desired_Px : Inport
  desired_Py : Inport  Port=2
  desired_Pz : Inport  Port=3
  actual_Px : Inport  Port=4
  actual_Py : Inport  Port=5
  actual_Pz : Inport  Port=6
  actual_Vx : Inport  Port=7
  actual_Vy : Inport  Port=8
  actual_Vz : Inport  Port=9
  actual_Az : Inport  Port=10
  Desired_Yaw : Inport  Port=11
  Band-limited Derivative{1..2,4,6,8..10} (7 alike) : TransferFcn  Numerator=[1 0]  Denominator=[0.1 1]
  Constant1 : Constant  Value=0.55
  Controllers 1 : Scope  NumInputPorts=9
  D_X : Gain  Gain=Kd_px
  D_X1 : Gain  Gain=Kd_vx
  D_X3 : Gain  Gain=Kd_py
  D_X4 : Gain  Gain=Kd_vy
  D_X6 : Gain  Gain=Kd_pz
  D_X7 : Gain  Gain=Kd_vz
  D_X8 : Gain  Gain=Kd_az
  Display : Display
  Display1 : Display
  I_X : Gain  Gain=Ki_px
  I_X1 : Gain  Gain=Ki_vx
  I_X3 : Gain  Gain=Ki_py
  I_X4 : Gain  Gain=Ki_vy
  I_X6 : Gain  Gain=Ki_pz
  I_X7 : Gain  Gain=Ki_vz
  I_X8 : Gain  Gain=Ki_az
  Integrator Limited{1,3..4,6} (4 alike) : Integrator  LimitOutput=on  UpperSaturationLimit=100  LowerSaturationLimit=-100
  Integrator Limited10 : Integrator  LimitOutput=on  UpperSaturationLimit=1000  LowerSaturationLimit=-1000
  Integrator Limited8 : Integrator  LimitOutput=on  UpperSaturationLimit=1000  LowerSaturationLimit=-1000
  Integrator Limited9 : Integrator  LimitOutput=on  UpperSaturationLimit=1000  LowerSaturationLimit=-1000
  Mux{,1,3..4,6..7} (6 alike) : Mux  Inputs=2
  Mux5 : Mux  Inputs=3
  P_X : Gain  Gain=Kp_px
  P_X1 : Gain  Gain=Kp_vx
  P_X3 : Gain  Gain=Kp_py
  P_X4 : Gain  Gain=Kp_vy
  P_X6 : Gain  Gain=Kp_pz
  P_X7 : Gain  Gain=Kp_vz
  P_X8 : Gain  Gain=Kp_az
  P_pr1 : Gain  Gain=-1
  Saturation : Saturate  UpperLimit=5  LowerLimit=-5
  Saturation1 : Saturate  UpperLimit=5  LowerLimit=-5
  Saturation2 : Saturate  UpperLimit=10  LowerLimit=0
  Sum{6,8,11,13,15..16,18} (7 alike) : Sum  Inputs=|+-
  Sum{4..5,7,12,17,19..20} (7 alike) : Sum  Inputs=++-
  Sum2 : Sum  Inputs=+|+
  accel2force : Gain  Gain=0.055
  roll_ctrl : Outport
  pitch_ctrl : Outport  Port=2
  yaw_ctrl : Outport  Port=3
  altura_ctrl : Outport  Port=4
  wires:
  Saturation1/1 -> roll_ctrl/1
  Saturation/1 -> pitch_ctrl/1
  P_pr1/1 -> Saturation1/1
  Mux7/1 -> Controllers 1/5
  Mux6/1 -> Controllers 1/4
  actual_Vy/1 -> Mux7/2, Sum13/2, Band-limited Derivative6/1
  desired_Py/1 -> Sum11/1, Mux6/1
  actual_Py/1 -> Mux6/2, Band-limited Derivative1/1, Sum11/2
  Constant1/1 -> Sum2/2
  accel2force/1 -> Sum2/1
  Sum2/1 -> Saturation2/1
  Sum19/1 -> accel2force/1
  Mux5/1 -> Controllers 1/9
  Mux4/1 -> Controllers 1/8
  Mux3/1 -> Controllers 1/7
  Sum17/1 -> Sum15/1, Mux5/1  "desired_Az"
  actual_Az/1 -> Sum15/2, Band-limited Derivative10/1, Mux5/2
  Sum20/1 -> Sum18/1, Mux4/1  "desired_Vz"
  actual_Vz/1 -> Band-limited Derivative9/1, Sum18/2, Mux4/2
  Mux1/1 -> Controllers 1/2
  Mux/1 -> Controllers 1/1
  I_X8/1 -> Sum19/2
  Band-limited Derivative10/1 -> D_X8/1
  D_X8/1 -> Sum19/3
  P_X8/1 -> Sum19/1
  Integrator Limited10/1 -> I_X8/1, Display/1
  Sum15/1 -> P_X8/1, Integrator Limited10/1
  I_X7/1 -> Sum17/2
  Band-limited Derivative9/1 -> D_X7/1
  D_X7/1 -> Sum17/3
  P_X7/1 -> Sum17/1
  Integrator Limited9/1 -> I_X7/1, Display1/1
  Sum18/1 -> Integrator Limited9/1, P_X7/1
  I_X6/1 -> Sum20/2
  desired_Pz/1 -> Sum16/1, Mux3/1
  Band-limited Derivative8/1 -> D_X6/1
  actual_Pz/1 -> Sum16/2, Band-limited Derivative8/1, Mux3/2
  D_X6/1 -> Sum20/3
  P_X6/1 -> Sum20/1
  Integrator Limited8/1 -> I_X6/1
  Sum16/1 -> P_X6/1, Integrator Limited8/1
  Sum12/1 -> Controllers 1/6, P_pr1/1  "desired_ROLL"
  Sum4/1 -> Mux7/1, Sum13/1  "desired_Vy"
  I_X4/1 -> Sum12/2
  Band-limited Derivative6/1 -> D_X4/1
  D_X4/1 -> Sum12/3
  P_X4/1 -> Sum12/1
  Integrator Limited6/1 -> I_X4/1
  Sum13/1 -> P_X4/1, Integrator Limited6/1
  I_X3/1 -> Sum4/2
  Band-limited Derivative1/1 -> D_X3/1
  D_X3/1 -> Sum4/3
  P_X3/1 -> Sum4/1
  Integrator Limited1/1 -> I_X3/1
  Sum11/1 -> Integrator Limited1/1, P_X3/1
  Sum7/1 -> Controllers 1/3, Saturation/1  "desired_PITCH"
  Sum5/1 -> Sum8/1, Mux1/1  "desired_Vx"
  I_X1/1 -> Sum7/2
  Band-limited Derivative4/1 -> D_X1/1
  actual_Vx/1 -> Band-limited Derivative4/1, Sum8/2, Mux1/2
  D_X1/1 -> Sum7/3
  P_X1/1 -> Sum7/1
  Integrator Limited4/1 -> I_X1/1
  Sum8/1 -> Integrator Limited4/1, P_X1/1
  Saturation2/1 -> altura_ctrl/1, Mux5/3
  I_X/1 -> Sum5/2
  desired_Px/1 -> Sum6/1, Mux/1
  Band-limited Derivative2/1 -> D_X/1
  actual_Px/1 -> Sum6/2, Band-limited Derivative2/1, Mux/2
  D_X/1 -> Sum5/3
  P_X/1 -> Sum5/1
  Integrator Limited3/1 -> I_X/1
  Sum6/1 -> P_X/1, Integrator Limited3/1
  Desired_Yaw/1 -> yaw_ctrl/1

== system quad_sim_mult_UAVs_coop_localization/Quadrotor 1/Quadrirrotor Communication ==
  roll : Inport
  pitch : Inport  Port=2
  yaw : Inport  Port=3
  throttle : Inport  Port=4
  Blank Message : robotlib/Blank Message  SourceLibraryInfo=This block requires Robotics System Toolbox  messageType=geometry_msgs/Quaternion  SampleTime=inf
      settings: SourceProductBaseCode=RO
  Bus Assignment1 : BusAssignment  DialogController=Simulink.DDGSource_BusAssignment  AssignedSignals=X,Y,Z,W
  Bus Selector1 : BusSelector  OutputSignals=Data
  Data Type Conversion : DataTypeConversion  OutDataTypeStr=double
  Multiport Selector : dspindex/Multiport Selector  rowsOrCols=Rows  idxCellArray={ 1,2,3,4,5,6,7,8,9}  idxErrMode=Generate Error
  Publish2 : robotlib/Publish  SourceLibraryInfo=This block requires Robotics System Toolbox  topicSource=Specify your own  topic=/commands_attitude_1  messageType=geometry_msgs/Quaternion  messageQueueLength=105
      settings: SourceProductBaseCode=RO
  Subscribe : robotlib/Subscribe  SourceLibraryInfo=This block requires Robotics System Toolbox  topicSource=Specify your own  topic=/quadrotor_states_1  messageType=std_msgs/Float32MultiArray  sampleTime=-1  messageQueueLength=51
      settings: SourceProductBaseCode=RO
  Terminator : Terminator
  quad_pos_x : Outport
  quad_pos_y : Outport  Port=2
  quad_pos_z : Outport  Port=3
  quad_vel_x : Outport  Port=4
  quad_vel_y : Outport  Port=5
  quad_vel_z : Outport  Port=6
  quad_acc_x : Outport  Port=7
  quad_acc_y : Outport  Port=8
  quad_acc_z : Outport  Port=9
  wires:
  roll/1 -> Bus Assignment1/2
  pitch/1 -> Bus Assignment1/3
  yaw/1 -> Bus Assignment1/4
  throttle/1 -> Bus Assignment1/5
  Bus Selector1/1 -> Data Type Conversion/1  "<Data>"
  Data Type Conversion/1 -> Multiport Selector/1
  Multiport Selector/9 -> quad_acc_z/1
  Multiport Selector/8 -> quad_acc_y/1
  Multiport Selector/7 -> quad_acc_x/1
  Multiport Selector/6 -> quad_vel_z/1
  Multiport Selector/5 -> quad_vel_y/1
  Multiport Selector/4 -> quad_vel_x/1
  Multiport Selector/3 -> quad_pos_z/1
  Multiport Selector/2 -> quad_pos_y/1
  Multiport Selector/1 -> quad_pos_x/1
  Bus Assignment1/1 -> Publish2/1
  Subscribe/2 -> Bus Selector1/1
  Subscribe/1 -> Terminator/1
  Blank Message/1 -> Bus Assignment1/1

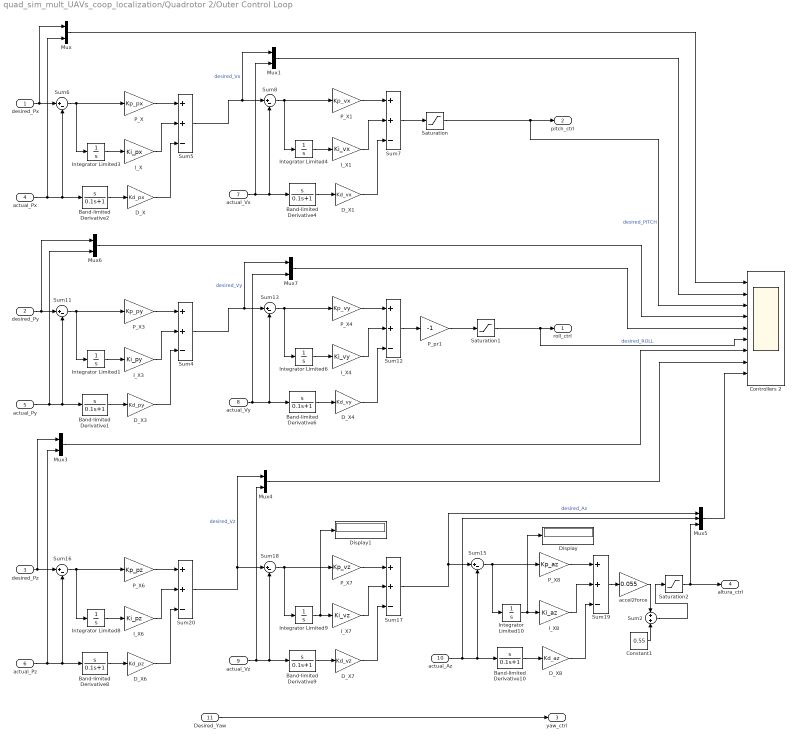
== system quad_sim_mult_UAVs_coop_localization/Quadrotor 2/Outer Control Loop ==
  desired_Px : Inport
  desired_Py : Inport  Port=2
  desired_Pz : Inport  Port=3
  actual_Px : Inport  Port=4
  actual_Py : Inport  Port=5
  actual_Pz : Inport  Port=6
  actual_Vx : Inport  Port=7
  actual_Vy : Inport  Port=8
  actual_Vz : Inport  Port=9
  actual_Az : Inport  Port=10
  Desired_Yaw : Inport  Port=11
  Band-limited Derivative{1..2,4,6,8..10} (7 alike) : TransferFcn  Numerator=[1 0]  Denominator=[0.1 1]
  Constant1 : Constant  Value=0.55
  Controllers 2 : Scope  NumInputPorts=9
  D_X : Gain  Gain=Kd_px
  D_X1 : Gain  Gain=Kd_vx
  D_X3 : Gain  Gain=Kd_py
  D_X4 : Gain  Gain=Kd_vy
  D_X6 : Gain  Gain=Kd_pz
  D_X7 : Gain  Gain=Kd_vz
  D_X8 : Gain  Gain=Kd_az
  Display : Display
  Display1 : Display
  I_X : Gain  Gain=Ki_px
  I_X1 : Gain  Gain=Ki_vx
  I_X3 : Gain  Gain=Ki_py
  I_X4 : Gain  Gain=Ki_vy
  I_X6 : Gain  Gain=Ki_pz
  I_X7 : Gain  Gain=Ki_vz
  I_X8 : Gain  Gain=Ki_az
  Integrator Limited{1,3..4,6} (4 alike) : Integrator  LimitOutput=on  UpperSaturationLimit=100  LowerSaturationLimit=-100
  Integrator Limited10 : Integrator  LimitOutput=on  UpperSaturationLimit=1000  LowerSaturationLimit=-1000
  Integrator Limited8 : Integrator  LimitOutput=on  UpperSaturationLimit=1000  LowerSaturationLimit=-1000
  Integrator Limited9 : Integrator  LimitOutput=on  UpperSaturationLimit=1000  LowerSaturationLimit=-1000
  Mux{,1,3..4,6..7} (6 alike) : Mux  Inputs=2
  Mux5 : Mux  Inputs=3
  P_X : Gain  Gain=Kp_px
  P_X1 : Gain  Gain=Kp_vx
  P_X3 : Gain  Gain=Kp_py
  P_X4 : Gain  Gain=Kp_vy
  P_X6 : Gain  Gain=Kp_pz
  P_X7 : Gain  Gain=Kp_vz
  P_X8 : Gain  Gain=Kp_az
  P_pr1 : Gain  Gain=-1
  Saturation : Saturate  UpperLimit=5  LowerLimit=-5
  Saturation1 : Saturate  UpperLimit=5  LowerLimit=-5
  Saturation2 : Saturate  UpperLimit=10  LowerLimit=0
  Sum{6,8,11,13,15..16,18} (7 alike) : Sum  Inputs=|+-
  Sum{4..5,7,12,17,19..20} (7 alike) : Sum  Inputs=++-
  Sum2 : Sum  Inputs=+|+
  accel2force : Gain  Gain=0.055
  roll_ctrl : Outport
  pitch_ctrl : Outport  Port=2
  yaw_ctrl : Outport  Port=3
  altura_ctrl : Outport  Port=4
  wires:
  Desired_Yaw/1 -> yaw_ctrl/1
  Sum6/1 -> Integrator Limited3/1, P_X/1
  Integrator Limited3/1 -> I_X/1
  P_X/1 -> Sum5/1
  D_X/1 -> Sum5/3
  actual_Px/1 -> Mux/2, Band-limited Derivative2/1, Sum6/2
  Band-limited Derivative2/1 -> D_X/1
  desired_Px/1 -> Mux/1, Sum6/1
  I_X/1 -> Sum5/2
  Saturation2/1 -> Mux5/3, altura_ctrl/1
  Sum8/1 -> P_X1/1, Integrator Limited4/1
  Integrator Limited4/1 -> I_X1/1
  P_X1/1 -> Sum7/1
  D_X1/1 -> Sum7/3
  actual_Vx/1 -> Mux1/2, Sum8/2, Band-limited Derivative4/1
  Band-limited Derivative4/1 -> D_X1/1
  I_X1/1 -> Sum7/2
  Sum5/1 -> Mux1/1, Sum8/1  "desired_Vx"
  Sum7/1 -> Saturation/1
  Sum11/1 -> P_X3/1, Integrator Limited1/1
  Integrator Limited1/1 -> I_X3/1
  P_X3/1 -> Sum4/1
  D_X3/1 -> Sum4/3
  Band-limited Derivative1/1 -> D_X3/1
  I_X3/1 -> Sum4/2
  Sum13/1 -> Integrator Limited6/1, P_X4/1
  Integrator Limited6/1 -> I_X4/1
  P_X4/1 -> Sum12/1
  D_X4/1 -> Sum12/3
  Band-limited Derivative6/1 -> D_X4/1
  I_X4/1 -> Sum12/2
  Sum4/1 -> Sum13/1, Mux7/1  "desired_Vy"
  Sum12/1 -> P_pr1/1
  Sum16/1 -> Integrator Limited8/1, P_X6/1
  Integrator Limited8/1 -> I_X6/1
  P_X6/1 -> Sum20/1
  D_X6/1 -> Sum20/3
  actual_Pz/1 -> Mux3/2, Band-limited Derivative8/1, Sum16/2
  Band-limited Derivative8/1 -> D_X6/1
  desired_Pz/1 -> Mux3/1, Sum16/1
  I_X6/1 -> Sum20/2
  Sum18/1 -> P_X7/1, Integrator Limited9/1
  Integrator Limited9/1 -> Display1/1, I_X7/1
  P_X7/1 -> Sum17/1
  D_X7/1 -> Sum17/3
  Band-limited Derivative9/1 -> D_X7/1
  I_X7/1 -> Sum17/2
  Sum15/1 -> Integrator Limited10/1, P_X8/1
  Integrator Limited10/1 -> Display/1, I_X8/1
  P_X8/1 -> Sum19/1
  D_X8/1 -> Sum19/3
  Band-limited Derivative10/1 -> D_X8/1
  I_X8/1 -> Sum19/2
  Mux/1 -> Controllers 2/1
  Mux1/1 -> Controllers 2/2
  actual_Vz/1 -> Mux4/2, Sum18/2, Band-limited Derivative9/1
  Sum20/1 -> Mux4/1, Sum18/1  "desired_Vz"
  actual_Az/1 -> Mux5/2, Band-limited Derivative10/1, Sum15/2
  Sum17/1 -> Mux5/1, Sum15/1  "desired_Az"
  Mux3/1 -> Controllers 2/7
  Mux4/1 -> Controllers 2/8
  Mux5/1 -> Controllers 2/9
  Sum19/1 -> accel2force/1
  Sum2/1 -> Saturation2/1
  accel2force/1 -> Sum2/1
  Constant1/1 -> Sum2/2
  actual_Py/1 -> Sum11/2, Band-limited Derivative1/1, Mux6/2
  desired_Py/1 -> Mux6/1, Sum11/1
  actual_Vy/1 -> Band-limited Derivative6/1, Sum13/2, Mux7/2
  Mux6/1 -> Controllers 2/4
  Mux7/1 -> Controllers 2/5
  P_pr1/1 -> Saturation1/1
  Saturation/1 -> Controllers 2/3, pitch_ctrl/1  "desired_PITCH"
  Saturation1/1 -> Controllers 2/6, roll_ctrl/1  "desired_ROLL"

== system quad_sim_mult_UAVs_coop_localization/Quadrotor 2/Quadrirrotor Communication ==
  roll : Inport
  pitch : Inport  Port=2
  yaw : Inport  Port=3
  throttle : Inport  Port=4
  Blank Message : robotlib/Blank Message  SourceLibraryInfo=This block requires Robotics System Toolbox  messageType=geometry_msgs/Quaternion  SampleTime=inf
      settings: SourceProductBaseCode=RO
  Bus Assignment1 : BusAssignment  DialogController=Simulink.DDGSource_BusAssignment  AssignedSignals=X,Y,Z,W
  Bus Selector1 : BusSelector  OutputSignals=Data
  Data Type Conversion : DataTypeConversion  OutDataTypeStr=double
  Multiport Selector : dspindex/Multiport Selector  rowsOrCols=Rows  idxCellArray={ 1,2,3,4,5,6,7,8,9}  idxErrMode=Generate Error
  Publish2 : robotlib/Publish  SourceLibraryInfo=This block requires Robotics System Toolbox  topicSource=Specify your own  topic=/commands_attitude_2  messageType=geometry_msgs/Quaternion  messageQueueLength=105
      settings: SourceProductBaseCode=RO
  Subscribe : robotlib/Subscribe  SourceLibraryInfo=This block requires Robotics System Toolbox  topicSource=Specify your own  topic=/quadrotor_states_2  messageType=std_msgs/Float32MultiArray  sampleTime=-1  messageQueueLength=51
      settings: SourceProductBaseCode=RO
  Terminator : Terminator
  quad_pos_x : Outport
  quad_pos_y : Outport  Port=2
  quad_pos_z : Outport  Port=3
  quad_vel_x : Outport  Port=4
  quad_vel_y : Outport  Port=5
  quad_vel_z : Outport  Port=6
  quad_acc_x : Outport  Port=7
  quad_acc_y : Outport  Port=8
  quad_acc_z : Outport  Port=9
  wires:
  Blank Message/1 -> Bus Assignment1/1
  Subscribe/1 -> Terminator/1
  Subscribe/2 -> Bus Selector1/1
  Bus Assignment1/1 -> Publish2/1
  Multiport Selector/1 -> quad_pos_x/1
  Multiport Selector/2 -> quad_pos_y/1
  Multiport Selector/3 -> quad_pos_z/1
  Multiport Selector/4 -> quad_vel_x/1
  Multiport Selector/5 -> quad_vel_y/1
  Multiport Selector/6 -> quad_vel_z/1
  Multiport Selector/7 -> quad_acc_x/1
  Multiport Selector/8 -> quad_acc_y/1
  Multiport Selector/9 -> quad_acc_z/1
  Data Type Conversion/1 -> Multiport Selector/1
  Bus Selector1/1 -> Data Type Conversion/1  "<Data>"
  throttle/1 -> Bus Assignment1/5
  yaw/1 -> Bus Assignment1/4
  pitch/1 -> Bus Assignment1/3
  roll/1 -> Bus Assignment1/2
